simulink library "mympclib"  (R2020a)
settings: Solver=VariableStepAuto  StartTime=0.0  StopTime=10.0  RelTol=1e-3
values from neighbouring files (symbols this model uses):
  Ts = 0.01    [calcCTSyetem.m]
undefined symbols (not defined in the file or in its folder): params, sysm
settings Model: Creator=kohei  LastModifiedBy=kohei

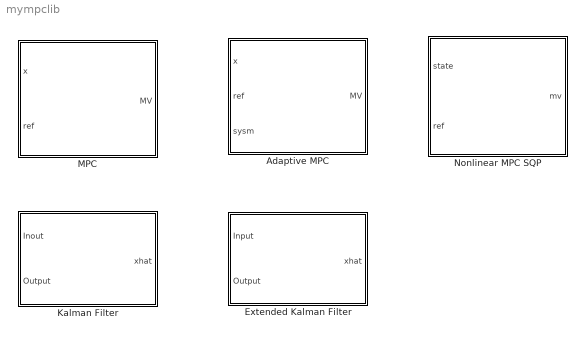
== system mympclib ==
  Adaptive MPC : Subsystem  TreatAsAtomicUnit=on  mask(Adaptive Model Predictive Control){params=params, numState=1, numRef=1, numMV=1, Ts=Ts, enableDist=off, numDist=1, enableSlack=off, enableStatus=off, enableMVseq=off}
      mask prompts: params "MPC Parameters"; numState "Dimension of State"; numRef "Dimension of Reference"; numMV "Dimension of Input"; Ts "Sampling time"; enableDist "Enable Disturbance Input"; numDist "Dimension of Disturbance"; enableSlack "Enable Slack Output"; enableStatus "Enable Status Output"; enableMVseq "Enable MVseq Output"
      mask help:
      | This is the Adaptive MPC (AMPC) Controller.
      | AMPC calculates the QP problem based on the linear plant model.
      | If you want to see the description, please push the help button.
      mask init:
      | numDist = initMaskPortMPC(numDist,enableDist,enableSlack,enableStatus,enableMVseq,'Adaptive MPC');
      | [params,~] = initMaskMPC(params,[],numState,numRef,numMV,numDist,'Adaptive MPC');
      | index = numState*params.PredictiveHorizon;
      | index2 = numMV*params.ControlHorizon;
      | index3 = numRef*params.PredictiveHorizon;
      | index4 = numMV*params.ControlHorizon+1;
      | index5 = 4*(numMV*params.ControlHorizon)+2*(numRef*params.PredictiveHorizon)+1;
      mask Help:
      | This block is the Adaptive MPC Controller.
      | AMPC calculates the QP problem based on the linear plant model.
      | 
      | >>Optimization formulation
      | -------------------------------------------------------------------------------------------------------------------------------------------------------------------
      | This MPC is formulated based on the next QP optimization.
      | 
      | J = 0.5 * ( (y - yref)'*Q*(y - yref) + du'*R*du + rho*slack^2 )
      | 
      | Subject to :
      | umin <= u <= umax
      | dumin <= du <= dumax
      | ymin - slack*vmin <= y <= ymax + slack*vmax
      | skack >= 0
      | 
      | One slack varable is introduced for relaxing the output constraint.
      | The vmin and vmax are the tunable parameter for relaxation which is able to specified by MPC parameter structure as "params.softConstRelaxation".
      | Please read the " Details of the parameter sturucture "params" and "sysm" ".
      | -------------------------------------------------------------------------------------------------------------------------------------------------------------------
      | 
      | >> Model Structure
      | -------------------------------------------------------------------------------------------------------------------------------------------------------------------
      | This block supports the discrete plant system as shown bellow:
      | Uppercase is indicated the Nominal value, Lowercase with 'd' suffix is indicated the perturbation.
      | 
      | State : x = X + dx
      | MV : u = U + du
      | Measurement Disturbance(MD) : md = MD + dmd
      | Output Value : y = Y +dy (dy = C*dx)
      | 
      | Model formulation :
      | dx(k+1) = A*dx(k)+ B*du(k) + Bd*dmd(k) + f0
      | y(K) = C*dx(K) + Y
      | 
      | Note : The direct feedthrough term "D" is not considered in this system.
      |           "f0" is the nominal value of the system at the operation point.
      | 
      | The plant model is streamed from the Input port "sysm" which is the Bus signal.
      | You need to define the Bus object named "sysBus" which includes A, B, Bd, C, f0 vector/matrix and the operation point of state, input, disturbance and output.
      | -------------------------------------------------------------------------------------------------------------------------------------------------------------------
      | 
      | >>Parameter
      | -------------------------------------------------------------------------------------------------------------------------------------------------------------------
      | The MPC parameter must be defined as structure variable.
      | And you must need to clarify the each dimension of "state", "ref", and "Input" and the Sampling time through mask dialog.
      | 
      | This block has four input ports "state", "ref", "md" and "sysm".
      | Where "n" is the order of state, "l" is the order of output value (OV), "m" is the order of manipulated variable (MV) and "nd" is the order of measurement disturbance (MD).
      | "state" : State variable of plant model (n×1)
      | "ref" : Reference for OV  (l×1)
      | "md" : Measurement Disturbance (nd×1)
      | "sysm" : Bus signal which includes the predictive model. The structuer of the Bus object is shown bellow :
      | 
      | sysm.A : A matrix
      | sysm.B : B matrix for MV
      | sysm.Bd : B matrix for MD
      | sysm.C : C matrix
      | sysm.U : Operation point of MV, Defalt : zeros(m,1)
      | sysm.MD : Operation point of MD, Default : zeros(nd,1)
      | sysm.Y : Operation point of OV, Default : zeros(l,1)
      | sysm.X : Operation point of state, Default : zeros(n,1)
      | sysm.f0: Operation point of system, Default : zeros(n,1)
      | 
      | You can create a Bus object automatically by uisng the API "createSysBusObject".
      | The API has four arguments 'n, m, nd, l'.
      | Example :
      | >sysBus = createSysBusObject(n,m,nd,l)
      | 
      | The output is four "mv" , "slack", "status" and "mvseq".
      | "mv" : Manipulated Variable which is optimized by MPC. (m×1)
      | "slack" : Slack variable for softening OV constrain. This value must be grater than 0 (>= 0).
      |              If the value is grater than 0, the OV constraint is softed to avoid infeasibe.
      | "status" : Status is for seeing whether or not feasible . If the value is "1", it means feasible, on the other hand the value is 0, it means infeasible.
      |                When the status is "0", the MPC applies a last MV for current step.
      | "mvseq": Sequence value of MV for futuer
      | -------------------------------------------------------------------------------------------------------------------------------------------------------------------
      | 
      | >>Solver
      | -------------------------------------------------------------------------------------------------------------------------------------------------------------------
      | You can choose two types solver for solving the QP.
      | First is the "Active set".
      | Second is the "Interior Point Method".
      | 
      | The Active set is appropriate to optimization class for small or middle size.
      | The Interior Point Method is appropriate to optimization class for large size.
      | 
      | Both default max iteration number is 50.
      | -------------------------------------------------------------------------------------------------------------------------------------------------------------------
      | 
      | >>Details of the parameter sturucture "params" and "sysm"
      | -------------------------------------------------------------------------------------------------------------------------------------------------------------------
      | The MPC parameter sturucture "params" must be configured as shown bellow :
      | Where "n" is the order of state, "l" is the order of OV, "m" is the order of MV and the "nd" is the order of MD.
      | 
      | params.Q : Weight of OV (l×l) , Default : Unit matrix
      | params.R : Weight of MV (m×m), Default : Unit matrix
      | params.PredictiveHorizon : Predictive horizon (Scalar), Default : 10
      | params.Controlhorizon : Control Horizon (Scalar), Default : 5
      | params.MV_max : MV max (m×1), Default : 999
      | params.MV_min : MV min (m×1), Default :  -999
      | params.dMV_max : Rate of MV max (m×1), Default : 999
      | params.dMV_min : Rate of MV min(m×1), Default : -999
      | params.OV_max : Rate of OV max (l×1), Default : 999
      | params.OV_min : Rate of OV min (l×1), Default : -999
      | params.rho : Weight of slack variable (Scalar), Default : 10^4
      | params.softConstRelaxation : Constant for OV relaxation by slack variable (l×1), Default : ones(l,1)
      | params.MV_scalefactor : Scale gain for MV (m×1), Default : ones(m,1)
      | params.OV_scalefactor : Scale gain for OV (l×1), Default : ones(m,1)
      | params.MD_scalefactor : Scale gain for MD (nd×1), Default : ones(m,1)
      | params.initialconditionMV : Initial value for MV (m×1), Default : ones(m,1)
      | params.SolverType :Scalar 1:= Active Set, 2:= Interior Point Method, Default : 1 (Active set)
      | params.IterationMax : Max iteration number of the QP solver, Default : 50
      | -------------------------------------------------------------------------------------------------------------------------------------------------------------------
      | 
      | >>Code generation
      | -------------------------------------------------------------------------------------------------------------------------------------------------------------------
      | Yes, support. If you have Simulink Coder and Embedded Coder, the implementation code can be generated from this block.
      | -------------------------------------------------------------------------------------------------------------------------------------------------------------------
      mask Callback enableDist:
      | enab = get_param(gcb,'enableDist');
      | 
      | % Set the 'MaskVisibilities' property for each parameters
      | if strcmp(enab,'on')
      |     set_param(gcb,'MaskVisibilities',{'on','on','on','on','on','on','on','on','on','on'});
      | else
      |     set_param(gcb,'MaskVisibilities',{'on','on','on','on','on','on','off','on','on','on'});
      | end
      mask Display:
      | fprintf('Adaptive MPC')
      | port_label('Output', 1, 'mv')
      | port_label('Input', 1, 'state')
      | port_label('Input', 2, 'ref')
      | port_label('Input', 3, 'sysm')
  Extended Kalman Filter : Subsystem  TreatAsAtomicUnit=on  mask(Extended Kalman filter){stateFunction=0, jacobianStateFunction=0, measurementFunction=0, jacobianMeasurmentFunction=0, Bv=0, Q=0, R=0, xhat0=0, P0=0, Ts=0, numState=0, numOutput=0, enableP=off, enableG=off}
      mask prompts: stateFunction "State Function"; jacobianStateFunction "Jacobian for the State Function"; measurementFunction "Measurment Function"; jacobianMeasurmentFunction "Jacobian for the Measurement Function"; Bv "Matrix for System noise v"; Q "Covariance matrix Q for system noise v"; R "Covariance matrix R for measurement noise w"; xhat0 "Initial value for xhat which is column vector"; P0 "Initial value for covariance matrix P"; Ts "Sampling time Ts"; numState "Order of state"; numOutput "Order of output"; enableP "Enable Covariance Marix output"; enableG "Enable Kalman Gain Matrix"
      mask help: This is the Extended Kalman filter(EKF) block.
      mask init:
      | p = initMaskEKF(stateFunction,measurementFunction,jacobianStateFunction,jacobianMeasurmentFunction);
      | initMaskPortKF(enableP,enableG,'EKF')
      mask Help:
      | This is the Extended Kalman filter(EKF) block.
      | Some parametrs are set through the mask diagram.
      | This block has two inputs named "Input" and "Output".
      | And it has three outputs named "xhat (Estimated state)", "P (Covariance matrix )" and "G (Kalman gain matrix )".
      | 
      | Support Formulation of EKF :
      | x(k+1) = f(x(k),u(k)) + Bv*v(k)
      | y(k) = h(x(k),u(k)) + w(k)
      | 
      | n : Order of state
      | m : Order of input
      | l : Order of output
      | 
      | f : Nonlinear dynamics function (n,1)
      | h : Nonlinear measurement function (l,1)
      | Bv : Gain matrix Bv for system noise v (n,n)
      | x : State (n,1)
      | u : Input (m,1)
      | v: System noise (n,1)
      | y : Output (l,1)
      | w : Measurement noise (l,1)
      | 
      | You need to prepare four MATLAB function and put them on the current folder or the MATLAB path.
      | Kind of the MATLAB function :
      | 
      | >Nonlinear discrete state function
      | 
      | >Jacobian of the Nonlinear state function about the state x with operate conditions x0 and u0.
      | 
      | >Nonlinear measurement function
      | 
      | >Jacobian of the Nonlinear measurement function about the state x with operate conditions x0 and u0.
      | 
      | Where, the above functions must be accepted three arguments x(state), u(input) and Ts(sampling time), and one output.
      | The order of three arguments has to be put as state, input and sampling time such like a below:
      | 
      | function out = fcn(x, u, Ts)
      | 
      | You have to set these function names through this mask dialog as the character array  by using sigle quotation.
      mask Display:
      | fprintf('Extended\n Kalman Filter')
      | port_label('Output', 1, 'xhat')
      | port_label('Input', 1, 'Input')
      | port_label('Input', 2, 'Output')
  Kalman Filter : Subsystem  TreatAsAtomicUnit=on  mask(Kalman filter){A=0, Bu=0, Bv=0, C=0, Q=0, R=0, xhat0=0, P0=0, Ts=0, enableP=off, enableG=off}
      mask prompts: A "System matrix A"; Bu "Input matrix Bu"; Bv "System noise matrix Bv"; C "Measurement matrix C"; Q "Covariance matrix for System noise v"; R "Covariance matrix for Measurement noise w"; xhat0 "Initial value for xhat which is column vector"; P0 "Initial value for covariance matrix P"; Ts "Sampling time Ts"; enableP "Enable Covariance Marix output"; enableG "Enable Kalman Gain Matrix"
      mask help: This is the LTI Kalman filter block.
      mask init:
      | initMaskPortKF(enableP,enableG,'KF')
      mask Help:
      | This is the LTI Kalman filter block.
      | All parametrs are set through the mask diagram.
      | This block has two inputs named "Input" and "Output".
      | And it has three outputs named "xhat (Estimated state)", "P (Covariance matrix )" and "G (Kalman gain matrix )".
      | 
      | Support Formulation of Kalman filter :
      | x(k+1) = A*x(k) + Bu*u(k) + Bv*v(k)
      | y(k) = C*x(k) + w(k)
      | 
      | A : System matrix A for state
      | Bu : System matrix Bu for input u
      | Bv : Gain matrix Bv for system noise v
      | C : System matrix C for output
      | x : State
      | u : Input
      | v : System noise
      | y : Output
      | w : Measurement noise
      mask Display:
      | fprintf('Kamlman Filter')
      | port_label('Output', 1, 'xhat')
      | port_label('Input', 1, 'Input')
      | port_label('Input', 2, 'Output')
  MPC : Subsystem  TreatAsAtomicUnit=on  mask(Model Predictive control){params=params, sysm=sysm, numState=1, numRef=1, numMV=1, Ts=Ts, enableDist=off, numDist=1, enableSlack=off, enableStatus=off, enableMVseq=off}
      mask prompts: params "MPC Parameters"; sysm "Control system"; numState "Dimension of State"; numRef "Dimension of Reference"; numMV "Dimension of MV"; Ts "Sampling time"; enableDist "Enable Disturbance Input"; numDist "Dimension of Disturbance"; enableSlack "Enable Slack Output"; enableStatus "Enable Status Output"; enableMVseq "Enable MVseq Output"
      mask help:
      | This is the MPC Controller.
      | MPC calculates the QP problem based on the linear plant model.
      | If you want to see the description, please push the help button.
      mask init:
      | numDist = initMaskPortMPC(numDist,enableDist,enableSlack,enableStatus,enableMVseq,'MPC');
      | [params,sysm] = initMaskMPC(params,sysm,numState,numRef,numMV,numDist,'MPC');
      | index = numState*params.PredictiveHorizon;
      | index2 = numMV*params.ControlHorizon;
      | index3 = numRef*params.PredictiveHorizon;
      | index4 = numMV*params.ControlHorizon+1;
      | index5 = 4*(numMV*params.ControlHorizon)+2*(numRef*params.PredictiveHorizon)+1;
      mask Help:
      | This block is the MPC Controller.
      | MPC calculates the QP problem based on the linear plant model.
      | 
      | >>Optimization formulation
      | -------------------------------------------------------------------------------------------------------------------------------------------------------------------
      | This MPC is formulated based on the next QP optimization.
      | 
      | J = 0.5 * ( (y - yref)'*Q*(y - yref) + du'*R*du + rho*slack^2 )
      | 
      | Subject to :
      | umin <= u <= umax
      | dumin <= du <= dumax
      | ymin - slack*vmin <= y <= ymax + slack*vmax
      | skack >= 0
      | 
      | One slack varable is introduced for releaxing the output constraint.
      | The vmin and vmax are tunable parameters for relaxation which are specified by the MPC parameter structure as "params.softConstRelaxation".
      | Please read the " Details of the parameter sturucture "params" and "sysm" ".
      | -------------------------------------------------------------------------------------------------------------------------------------------------------------------
      | 
      | 
      | >> Model Structure
      | -------------------------------------------------------------------------------------------------------------------------------------------------------------------
      | This block supports the discrete plant system as shown bellow:
      | Uppercase is indicated the Nominal value, Lowercase with 'd' suffix is indicated the perturbation.
      | 
      | State : x = X + dx
      | MV : u = U + du
      | Measurement Disturbance(MD) : md = MD + dmd
      | Output Value : y = Y +dy (dy = C*dx)
      | 
      | Model formulation :
      | dx(k+1) = A*dx(k)+ B*du(k) + Bd*dmd(k) + f0
      | y(K) = C*dx(K) + Y
      | 
      | Note : The direct feedthrough term "D" is not considered in this system.
      |           "f0" is the nominal value of the system at the operation point.
      | -------------------------------------------------------------------------------------------------------------------------------------------------------------------
      | 
      | 
      | >>Parameter
      | -------------------------------------------------------------------------------------------------------------------------------------------------------------------
      | The MPC parameter and the Control system must be defined as a structure variable.
      | The Sampling time must be set through mask dialog.
      | 
      | This block has three input ports "state", "ref" and "md".
      | Where, "n" is the order of state, "l" is the order of Output value (OV),  "m" is the order of Manipulated variable (MV) and "nd" is the order of measurment disturbance (MD).
      | "state" : State variable of plant model (n×1)
      | "ref" : Reference for OV  (l×1)
      | "md" : Measurement Disturbance (nd×1)
      | 
      | The output is three "mv" , "slack" and "status".
      | "MV" : Manipulated Variable which is optimized by MPC. (m×1)
      | "slack" : Slack variable for softening OV constrain. This value must be grater than 0 (>= 0).
      |              If the value is grater than 0, the OV constraint is softed to avoid infeasibe.
      | "status" : Status is for seeing whether or not feasible. If the value is "1", it means feasible, on the other hand the value is "0", it means infeasible.
      |                When the status is "0", the MPC applies a last MV for current step.
      | "mvseq": Sequence value of MV for futuer
      | -------------------------------------------------------------------------------------------------------------------------------------------------------------------
      | 
      | >>Solver
      | -------------------------------------------------------------------------------------------------------------------------------------------------------------------
      | You can choose two types solver for solving the QP.
      | First is the "Active set".
      | Second is the "Interior Point Method".
      | 
      | The Active set is appropriate to optimization class for small or middle size.
      | The Interior Point Method is appropriate to optimization class for large size.
      | 
      | Both default max iteration number is 50.
      | -------------------------------------------------------------------------------------------------------------------------------------------------------------------
      | 
      | >>Details of the parameter sturucture "params" and "sysm"
      | -------------------------------------------------------------------------------------------------------------------------------------------------------------------
      | The MPC parameter sturucture "params" must be configured as shown bellow :
      | Where the "n" is the order of state, "l" is the order of OV, "m" is the order of MV and the "nd" is the order of MD.
      | 
      | params.Q : Weight of OV (l×l) , Default : Unit matrix
      | params.R : Weight of MV (m×m), Default : Unit matrix
      | params.PredictiveHorizon : Predictive horizon (Scalar), Default : 10
      | params.Controlhorizon : Control Horizon (Scalar), Default : 5
      | params.MV_max : MV max (m×1), Default : 999
      | params.MV_min : MV min (m×1), Default :  -999
      | params.dMV_max : Rate of MV max (m×1), Default : 999
      | params.dMV_min : Rate of MV min(m×1), Default : -999
      | params.OV_max : Rate of OV max (l×1), Default : 999
      | params.OV_min : Rate of OV min (l×1), Default : -999
      | params.rho : Weight of slack variable (Scalar), Default : 10^4
      | params.softConstRelaxation : Constant for OV relaxation by slack variable (l×1), Default : ones(l,1)
      | params.MV_scalefactor : Scale gain for MV (m×1), Default : ones(m,1)
      | params.OV_scalefactor : Scale gain for OV (l×1), Default : ones(m,1)
      | params.MD_scalefactor : Scale gain for MD (nd×1), Default : ones(m,1)
      | params.initialconditionMV : Initial value for MV (m×1), Default : ones(m,1)
      | params.SolverType :Scalar, 1:= Active Set, 2:= Interior Point Method, Default : 1 (Active set)
      | params.IterationMax : Max iteration number of the QP solver, Default : 50
      | 
      | The Control system sturucture "syms" must be includes bellow items :
      | sysm.A : A matrix
      | sysm.B : B matrix for MV
      | sysm.Bd : B matrix for MD
      | sysm.C : C matrix
      | sysm.U : Operation point of MV, Defalt : zeros(m,1)
      | sysm.MD : Operation point of MD, Default : zeros(nd,1)
      | sysm.Y : Operation point of OV, Default : zeros(l,1)
      | sysm.X : Operation point of state, Default : zeros(n,1)
      | sysm.f0: Operation point of system, Default : zeros(n,1)
      | -------------------------------------------------------------------------------------------------------------------------------------------------------------------
      | 
      | >>Code generation
      | -------------------------------------------------------------------------------------------------------------------------------------------------------------------
      | Yes, support. If you have Simulink Coder and Embedded Coder, the implementation code can be generated from this block.
      | -------------------------------------------------------------------------------------------------------------------------------------------------------------------
      mask Callback enableDist:
      | enab = get_param(gcb,'enableDist');
      | 
      | % Set the 'MaskVisibilities' property for each parameters
      | if strcmp(enab,'on')
      |     set_param(gcb,'MaskVisibilities',{'on','on','on','on','on','on','on','on','on','on','on'});
      | else
      |     set_param(gcb,'MaskVisibilities',{'on','on','on','on','on','on','on','off','on','on','on'});
      | end
      mask Display:
      | fprintf('MPC')
      | port_label('Output', 1, 'mv')
      | port_label('Input', 1, 'state')
      | port_label('Input', 2, 'ref')
  Nonlinear MPC SQP : Subsystem  TreatAsAtomicUnit=on  mask(Nonlinear Model Predictive Control){params=params, nx=0, ny=0, nu=0, Ts=0, enableDist=off, nd=0, enableSlack=off, enableStatus=off}
      mask prompts: params "MPC Parameters"; nx "Dimension of State"; ny "Dimension of Output"; nu "Dimension of Input"; Ts "Sampling time"; enableDist "Enable Disturbance Input"; nd "Dimension of Disturbance"; enableSlack "Enable Slack Output"; enableStatus "Enable Status Output"
      mask help:
      | This is the NMPC Controller.
      | Calculate the NP problem by using the fmincon solver with SQP.
      |
      | Note :
      | "fmincon" is a builtin command of the Optimization Toolbox.
      | You need to install this toolbox for run this block.
      |
      | If you want to see the description, please push the help button.
      mask init:
      | nd = initMaskPortNMPC(nd,enableDist,enableSlack,enableStatus,'SQP');
      | params = initMaskNMPC(params,nx,ny,nu,nd);
      | mv0 = params.initialconditionMV;
      | x0 = params.initialconditionState;
      | Hp = params.PredictiveHorizon;
      | Hc = params.ControlHorizon;
      | d0 = [kron(ones(Hc,1),mv0);0];
      mask Help:
      | This block is the Nonlinear MPC Controller.
      | Calculate the NP problem by using the fmincon solver with SQP.
      | Note : "fmincon" is a builtin command of the Optimization Toolbox. You need to install this toolbox for run this block.
      | 
      | >>Optimization formulation
      | -------------------------------------------------------------------------------------------------------------------------------------------------------------------
      | This MPC is formulated based on the next QP optimization.
      | 
      | J = 0.5 * ( (y - yref)'*Q*(y - yref) + u'*R*u + rho*slack^2 )
      | 
      | Subject to :
      | umin <= u <= umax
      | dumin <= du <= dumax
      | ymin - slack*vmin <= y <= ymax + slack*vmax
      | skack >= 0
      | 
      | One slack varable is introduced for relaxing the output constraint.
      | The vmin and vmax are the tunable parameter for relaxation which is able to specified by MPC parameter structure as "params.softConstRelaxation".
      | Please read the " Details of the parameter sturucture "params"' and "sysm" ".
      | -------------------------------------------------------------------------------------------------------------------------------------------------------------------
      | 
      | 
      | >> Model Structure
      | -------------------------------------------------------------------------------------------------------------------------------------------------------------------
      | This block supports the discrete nonlinear plant system as shown bellow:
      | 
      | Model formulation :
      | dx(k+1) = f( x(k), u(k) ,d(k) )
      | y(K) = h( x(k), u(k) )
      | 
      | The "f" is the state function and the "h" is the measurement function.
      | These are defined by MATLAB Function.
      | -------------------------------------------------------------------------------------------------------------------------------------------------------------------
      | 
      | >>Parameter
      | -------------------------------------------------------------------------------------------------------------------------------------------------------------------
      | The MPC parameter must be defined as structure variable.
      | And you must need to clarify the each dimension of "State", "Output", "Input" and Sampling time through mask dialog.
      | 
      | This block has three input ports "state", "ref", and "md".
      | Where "n" is the order of state, "l" is the order of output value (OV),  "m" is the order of manipulated variable (MV) and "nd" is the order of measurement disturbance (MD).
      | "state" : State variable of plant model (n×1)
      | "ref" : Reference for OV  (l×1)
      | "md" : Measurement Disturbance (nd×1)
      | 
      | The output is three "mv" , "slack", and "status".
      | "mv" : Manipulated Variable which is optimized by MPC. (m×1)
      | "slack" : Slack variable for softening OV constraint. This value must be grater than 0 (>= 0).
      |              If the value is grater than 0, the OV constraint is softed to avoid infeasibe solution.
      | "status" : Status is for seeing whether or not feasible. If the value is "1", it means feasible, on the other hand the value is 0, it means infeasible.
      |                When the value equals "0", the MPC applies a last MV for current step.
      | -------------------------------------------------------------------------------------------------------------------------------------------------------------------
      | 
      | >>Solver
      | -------------------------------------------------------------------------------------------------------------------------------------------------------------------
      | NMPC block is implemented by using the "fmincon".
      | And for solving NP problem, SQP algorithm is used.
      | The "fmincon" is builtin command of the Optimization Toolbox.
      | So, you need to install the toolbox in your machine.
      | Default max iteration number is 50 times.
      | -------------------------------------------------------------------------------------------------------------------------------------------------------------------
      | 
      | >>Details of the parameter sturucture "params".
      | -------------------------------------------------------------------------------------------------------------------------------------------------------------------
      | The MPC parameter sturucture "params" must be configured as shown bellow :
      | Where "n" is the order of state, "l" is the order of OV, "m" is the order of MV.
      | 
      | params.stateFunction : Function name for the state evolution
      | params.measurementFunction : Function name for the measurement
      | params.Q : Weight of OV (l×l) , Default : Unit matrix
      | params.R : Weight of MV (m×m), Default : Unit matrix
      | params.PredictiveHorizon : Predictive horizon (Scalar), Default : 10
      | params.Controlhorizon : Control Horizon (Scalar), Default : 5
      | params.MV_max : MV max (m×1), Default : 999
      | params.MV_min : MV min (m×1), Default :  -999
      | params.dMV_max : Rate of MV max (m×1), Default : 999
      | params.dMV_min : Rate of MV min(m×1), Default : -999
      | params.OV_max : Rate of OV max (l×1), Default : 999
      | params.OV_min : Rate of OV min (l×1), Default : -999
      | params.rho : Weight of slack variable (Scalar), Default : 10^4
      | params.softConstRelaxation : Constant for OV relaxation by slack variable (l×1), Default : ones(l,1)
      | params.MV_scalefactor : Scale gain for MV (m×1), Default : ones(m,1)
      | params.OV_scalefactor : Scale gain for OV (l×1), Default : ones(m,1)
      | params.initialconditionMV : Initial value for MV (m×1), Default : zeros(m,1)
      | params.initialconditionState : Initial value for State (n×1), Default : zeros(m,1)
      | params.IterationMax : Max iteration number of the solver, Default : 50
      | -------------------------------------------------------------------------------------------------------------------------------------------------------------------
      | 
      | >>Code generation
      | -------------------------------------------------------------------------------------------------------------------------------------------------------------------
      | Yes, support. If you have Simulink Coder and Embedded Coder, the implementation code can be generated from this block.
      | -------------------------------------------------------------------------------------------------------------------------------------------------------------------
      mask Callback enableStatus:
      | enab = get_param(gcb,'enableDist');
      | 
      | % Set the 'MaskVisibilities' property for each parameters
      | if strcmp(enab,'on')
      |     set_param(gcb,'MaskVisibilities',{'on','on','on','on','on','on','on','on','on'});
      | else
      |     set_param(gcb,'MaskVisibilities',{'on','on','on','on','on','on','off','on','on'});
      | end
      mask Display:
      | fprintf('Nonlinear MPC\nSQP')
      | port_label('Output', 1, 'mv')
      | port_label('Input', 1, 'state')
      | port_label('Input', 2, 'ref')

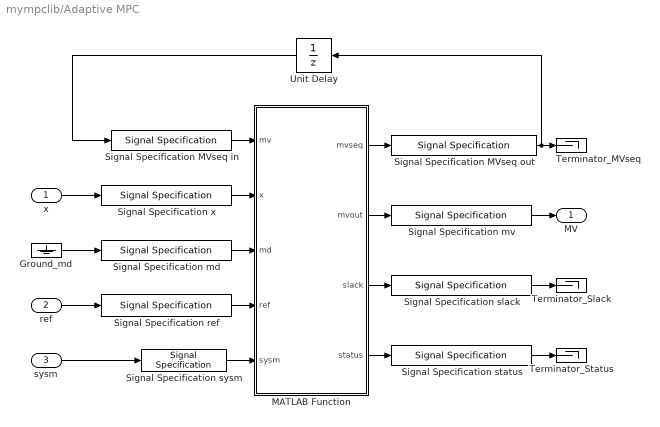
== system mympclib/Adaptive MPC ==
  x : Inport
  ref : Inport  Port=2
  sysm : Inport  Port=3
  Ground_md : Ground
  MATLAB Function : MATLAB Function  TreatAsAtomicUnit=on  SystemSampleTime=Ts
  Signal Specification MVseq in : SignalSpecification  OutDataTypeStr=double  Dimensions=index2  SampleTime=Ts
  Signal Specification MVseq out : SignalSpecification  OutDataTypeStr=double  Dimensions=index2  SampleTime=Ts
  Signal Specification md : SignalSpecification  OutDataTypeStr=double  Dimensions=numDist  SampleTime=Ts
  Signal Specification mv : SignalSpecification  OutDataTypeStr=double  Dimensions=numMV  SampleTime=Ts
  Signal Specification ref : SignalSpecification  OutDataTypeStr=double  Dimensions=numRef  SampleTime=Ts
  Signal Specification slack : SignalSpecification  OutDataTypeStr=double  Dimensions=1  SampleTime=Ts
  Signal Specification status : SignalSpecification  OutDataTypeStr=boolean  Dimensions=1  SampleTime=Ts
  Signal Specification sysm : SignalSpecification  SampleTime=Ts
  Signal Specification x : SignalSpecification  OutDataTypeStr=double  Dimensions=numState  SampleTime=Ts
  Terminator_MVseq : Terminator
  Terminator_Slack : Terminator
  Terminator_Status : Terminator
  Unit Delay : UnitDelay  InitialCondition=kron(ones(params.ControlHorizon,1) , params.initialconditionMV)  SampleTime=-1  HasFrameUpgradeWarning=on
  MV : Outport
  wires:
  MATLAB Function/3(slack) -> Signal Specification slack/1
  MATLAB Function/4(status) -> Signal Specification status/1
  x/1 -> Signal Specification x/1
  ref/1 -> Signal Specification ref/1
  Signal Specification x/1 -> MATLAB Function/2(x)
  Signal Specification md/1 -> MATLAB Function/3(md)
  Signal Specification ref/1 -> MATLAB Function/4(ref)
  sysm/1 -> Signal Specification sysm/1
  MATLAB Function/2(mvout) -> Signal Specification mv/1
  Signal Specification sysm/1 -> MATLAB Function/5(sysm)
  MATLAB Function/1(mvseq) -> Signal Specification MVseq out/1
  Unit Delay/1 -> Signal Specification MVseq in/1
  Signal Specification mv/1 -> MV/1
  Signal Specification MVseq in/1 -> MATLAB Function/1(mv)
  Signal Specification MVseq out/1 -> Unit Delay/1, Terminator_MVseq/1
  Signal Specification slack/1 -> Terminator_Slack/1
  Signal Specification status/1 -> Terminator_Status/1
  Ground_md/1 -> Signal Specification md/1

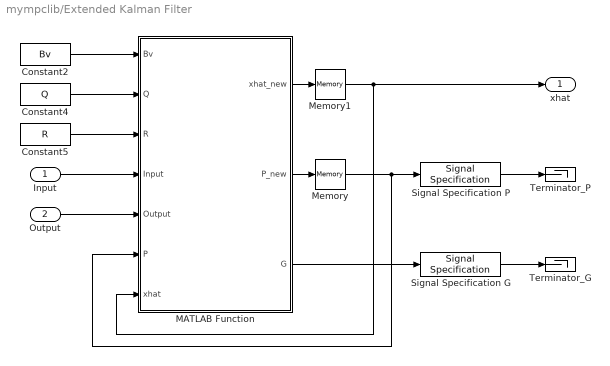
== system mympclib/Extended Kalman Filter ==
  Input : Inport
  Output : Inport  Port=2
  Constant2 : Constant  Value=Bv
  Constant4 : Constant  Value=Q
  Constant5 : Constant  Value=R
  MATLAB Function : MATLAB Function  TreatAsAtomicUnit=on  SystemSampleTime=Ts
  Memory : Memory  InitialCondition=P0  InheritSampleTime=on  LinearizeMemory=on  LinearizeAsDelay=on
  Memory1 : Memory  InitialCondition=xhat0  InheritSampleTime=on  LinearizeMemory=on  LinearizeAsDelay=on
  Signal Specification G : SignalSpecification  SampleTime=Ts
  Signal Specification P : SignalSpecification  SampleTime=Ts
  Terminator_G : Terminator
  Terminator_P : Terminator
  xhat : Outport
  wires:
  Constant2/1 -> MATLAB Function/1(Bv)
  MATLAB Function/3(G) -> Signal Specification G/1
  Constant5/1 -> MATLAB Function/3(R)
  Memory1/1 -> xhat/1, MATLAB Function/7(xhat)
  MATLAB Function/2(P_new) -> Memory/1
  MATLAB Function/1(xhat_new) -> Memory1/1
  Input/1 -> MATLAB Function/4(Input)
  Output/1 -> MATLAB Function/5(Output)
  Constant4/1 -> MATLAB Function/2(Q)
  Memory/1 -> Signal Specification P/1, MATLAB Function/6(P)
  Signal Specification P/1 -> Terminator_P/1
  Signal Specification G/1 -> Terminator_G/1

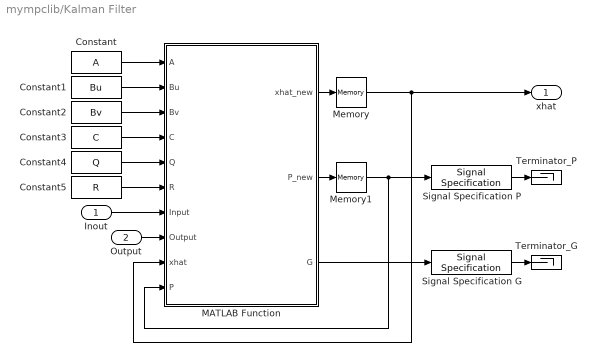
== system mympclib/Kalman Filter ==
  Inout : Inport
  Output : Inport  Port=2
  Constant : Constant  Value=A
  Constant1 : Constant  Value=Bu
  Constant2 : Constant  Value=Bv
  Constant3 : Constant  Value=C
  Constant4 : Constant  Value=Q
  Constant5 : Constant  Value=R
  MATLAB Function : MATLAB Function  TreatAsAtomicUnit=on  SystemSampleTime=Ts
  Memory : Memory  InitialCondition=xhat0  InheritSampleTime=on  LinearizeMemory=on  LinearizeAsDelay=on
  Memory1 : Memory  InitialCondition=P0  InheritSampleTime=on  LinearizeMemory=on  LinearizeAsDelay=on
  Signal Specification G : SignalSpecification  SampleTime=Ts
  Signal Specification P : SignalSpecification  SampleTime=Ts
  Terminator_G : Terminator
  Terminator_P : Terminator
  xhat : Outport
  wires:
  MATLAB Function/3(G) -> Signal Specification G/1
  Constant1/1 -> MATLAB Function/2(Bu)
  MATLAB Function/2(P_new) -> Memory1/1
  MATLAB Function/1(xhat_new) -> Memory/1
  Constant5/1 -> MATLAB Function/6(R)
  Inout/1 -> MATLAB Function/7(Input)
  Constant2/1 -> MATLAB Function/3(Bv)
  Constant3/1 -> MATLAB Function/4(C)
  Constant/1 -> MATLAB Function/1(A)
  Output/1 -> MATLAB Function/8(Output)
  Constant4/1 -> MATLAB Function/5(Q)
  Memory/1 -> MATLAB Function/9(xhat), xhat/1
  Memory1/1 -> MATLAB Function/10(P), Signal Specification P/1
  Signal Specification P/1 -> Terminator_P/1
  Signal Specification G/1 -> Terminator_G/1

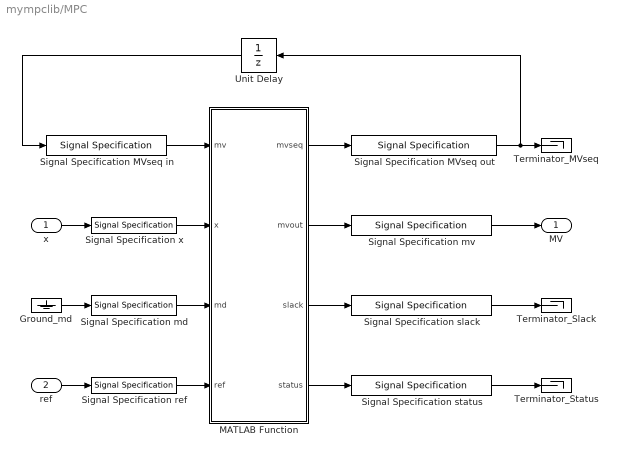
== system mympclib/MPC ==
  x : Inport
  ref : Inport  Port=2
  Ground_md : Ground
  MATLAB Function : MATLAB Function  TreatAsAtomicUnit=on  SystemSampleTime=Ts
  Signal Specification MVseq in : SignalSpecification  OutDataTypeStr=double  Dimensions=index2  SampleTime=Ts
  Signal Specification MVseq out : SignalSpecification  OutDataTypeStr=double  Dimensions=index2  SampleTime=Ts
  Signal Specification md : SignalSpecification  Dimensions=numDist  SampleTime=Ts
  Signal Specification mv : SignalSpecification  OutDataTypeStr=double  Dimensions=numMV  SampleTime=Ts
  Signal Specification ref : SignalSpecification  Dimensions=numRef  SampleTime=Ts
  Signal Specification slack : SignalSpecification  OutDataTypeStr=double  Dimensions=1  SampleTime=Ts
  Signal Specification status : SignalSpecification  OutDataTypeStr=boolean  Dimensions=1  SampleTime=Ts
  Signal Specification x : SignalSpecification  Dimensions=numState  SampleTime=Ts
  Terminator_MVseq : Terminator
  Terminator_Slack : Terminator
  Terminator_Status : Terminator
  Unit Delay : UnitDelay  InitialCondition=kron(ones(params.ControlHorizon,1) , params.initialconditionMV)  SampleTime=-1  HasFrameUpgradeWarning=on
  MV : Outport
  wires:
  Signal Specification ref/1 -> MATLAB Function/4(ref)
  Signal Specification md/1 -> MATLAB Function/3(md)
  Signal Specification x/1 -> MATLAB Function/2(x)
  ref/1 -> Signal Specification ref/1
  x/1 -> Signal Specification x/1
  MATLAB Function/4(status) -> Signal Specification status/1
  MATLAB Function/3(slack) -> Signal Specification slack/1
  MATLAB Function/2(mvout) -> Signal Specification mv/1
  Signal Specification MVseq in/1 -> MATLAB Function/1(mv)
  MATLAB Function/1(mvseq) -> Signal Specification MVseq out/1
  Signal Specification mv/1 -> MV/1
  Signal Specification MVseq out/1 -> Unit Delay/1, Terminator_MVseq/1
  Unit Delay/1 -> Signal Specification MVseq in/1
  Ground_md/1 -> Signal Specification md/1
  Signal Specification slack/1 -> Terminator_Slack/1
  Signal Specification status/1 -> Terminator_Status/1

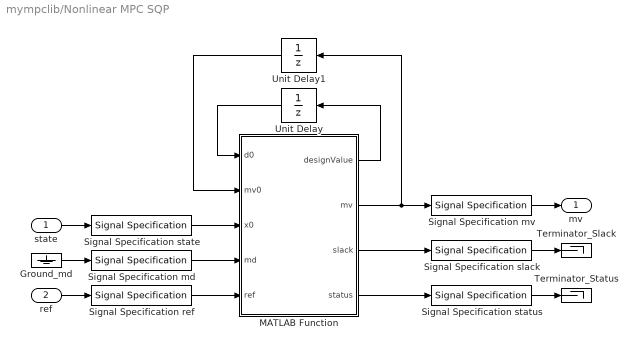
== system mympclib/Nonlinear MPC SQP ==
  state : Inport
  ref : Inport  Port=2
  Ground_md : Ground
  MATLAB Function : MATLAB Function  TreatAsAtomicUnit=on  SystemSampleTime=Ts
  Signal Specification md : SignalSpecification  OutDataTypeStr=double  Dimensions=nd  SampleTime=Ts
  Signal Specification mv : SignalSpecification  OutDataTypeStr=double  Dimensions=nu  SampleTime=Ts
  Signal Specification ref : SignalSpecification  OutDataTypeStr=double  Dimensions=ny  SampleTime=Ts
  Signal Specification slack : SignalSpecification  OutDataTypeStr=double  Dimensions=1  SampleTime=Ts
  Signal Specification state : SignalSpecification  OutDataTypeStr=double  Dimensions=nx  SampleTime=Ts
  Signal Specification status : SignalSpecification  OutDataTypeStr=boolean  Dimensions=1  SampleTime=Ts
  Terminator_Slack : Terminator
  Terminator_Status : Terminator
  Unit Delay : UnitDelay  InitialCondition=d0  SampleTime=Ts  HasFrameUpgradeWarning=on
  Unit Delay1 : UnitDelay  InitialCondition=mv0  SampleTime=Ts  HasFrameUpgradeWarning=on
  mv : Outport
  wires:
  state/1 -> Signal Specification state/1
  MATLAB Function/2(mv) -> Signal Specification mv/1, Unit Delay1/1
  MATLAB Function/1(designValue) -> Unit Delay/1
  Unit Delay/1 -> MATLAB Function/1(d0)
  ref/1 -> Signal Specification ref/1
  MATLAB Function/4(status) -> Signal Specification status/1
  MATLAB Function/3(slack) -> Signal Specification slack/1
  Unit Delay1/1 -> MATLAB Function/2(mv0)
  Signal Specification state/1 -> MATLAB Function/3(x0)
  Signal Specification md/1 -> MATLAB Function/4(md)
  Signal Specification ref/1 -> MATLAB Function/5(ref)
  Signal Specification mv/1 -> mv/1
  Ground_md/1 -> Signal Specification md/1
  Signal Specification slack/1 -> Terminator_Slack/1
  Signal Specification status/1 -> Terminator_Status/1

== matlab function mympclib/Nonlinear MPC SQP/MATLAB Function ==
  data: d0 input; mv0 input; designValue output; x0 input; md input; ref input; mv output; slack output; status output; params parameter; ny parameter; nu parameter; nx parameter
function [designValue,mv,slack,status] = fcn(d0,mv0,x0,md,ref,params,ny,nu,nx)
% Wraper for the nmpcfcn

% Initialization
designValue = zeros(length(d0),1,'like',d0);
mv = zeros(length(mv0),1,'like',mv0);
slack = zeros(1);
status = false;

[designValue,mv,slack,status] = nmpcfcn(d0,x0,mv0,md,ref,params,ny,nu,nx);
end
%EOF

== matlab function mympclib/Kalman Filter/MATLAB Function ==
  data: A input; xhat_new output; Bu input; Bv input; C input; Q input; R input; Input input; Output input; xhat input; P input; P_new output; G output
function [xhat_new,P_new,G] = fcn(A,Bu,Bv,C,Q,R,Input,Output,xhat,P)
%#codegen
% Wrapper function for Kalman filter function kf

% Initialization
n = size(A,1);
l = length(Output);
xhat_new = zeros(n,1);
P_new = zeros(n);
G = zeros(n,l);

% Call kf fucntion
[xhat_new,P_new,G] = kf(A,Bu,Bv,C,Q,R,Input,Output,xhat,P);
end
%EOF

== matlab function mympclib/MPC/MATLAB Function ==
  data: mvseq output; mv input; x input; mvout output; md input; ref input; slack output; status output boolean; params parameter; sysm parameter; index parameter size=1; index2 parameter size=1; index3 parameter size=1; index4 parameter size=1; index5 parameter size=1
function [mvseq,mvout,slack,status] = fcn(mv,x,md,ref,params,sysm,index,index2,index3,index4,index5)
% Wrapper of "mpcfcn"
% x:Output value(OV)
% d:Disturbance
% ref:Reference for OV
% sysm:Construnstion of system(A,B,C,D)
% params:MPC parameter constructs
% Dimenstions of each matrix:
% index = n*Hp
% index2 = m*Hc
% index3 = l*Hp
% index4 = (m*Hc)+1
% index5 = (4*index2)+(2*index3)+1
% Initlialization of outputs

% coder.extrinsic('mpcfcn');

% Initlialization of outputs
m = size(sysm.B,2);
slack = zeros(1);
status = false;
mvseq = zeros(index2,1);
mvout = zeros(m,1);

% Call mpcfcn
[mvopt,slack,status] = mpcfcn(x,mv,md,ref,sysm,params,index,index2,index3,index4,index5);
mvout = mvopt(1:m,1);
mvseq = mvopt;
%EOF

== matlab function mympclib/Adaptive MPC/MATLAB Function ==
  data: mvseq output; mv input; x input; mvout output; md input; ref input; slack output; status output boolean; params parameter; sysm input; index parameter size=1; index2 parameter size=1; index3 parameter size=1; index4 parameter size=1; index5 parameter size=1
function [mvseq,mvout,slack,status] = fcn(mv,x,md,ref,params,sysm,index,index2,index3,index4,index5)
% Wrapper of "mpcfcn"
% x:Output value(OV)
% d:Disturbance
% ref:Reference for OV
% sysm:Construnstion of system(A,B,C,D)
% params:MPC parameter constructs
% Dimenstions of each matrix:
% index = n*Hp
% index2 = m*Hc
% index3 = l*Hp
% index4 = (m*Hc)+1
% index5 = (4*index2)+(2*index3)+1

% Initlialization of outputs
m = size(sysm.B,2);
slack = zeros(1);
status = false;
mvseq = zeros(index2,1);
mvout = zeros(m,1);

% Call mpcfcn
[mvopt,slack,status] = mpcfcn(x,mv,md,ref,sysm,params,index,index2,index3,index4,index5);
mvout = mvopt(1:m,1);
mvseq = mvopt;
%EOF

== matlab function mympclib/Extended Kalman Filter/MATLAB Function ==
  data: xhat_new output; Bv input; Q input; R input; Input input; Output input; P input; xhat input; P_new output; G output; numState parameter; numOutput parameter; Ts parameter; p parameter
function [xhat_new,P_new,G] = fcn(Bv,Q,R,Input,Output,P,xhat,numState,numOutput,Ts,p)
%#codegen
% Wrapper function for Extended Kalman filter function ekf

% Initialization
n = numState;
l = numOutput;
xhat_new = zeros(n,1);
P_new = zeros(n);
G = zeros(n,l);

% Function handle
f = str2func(p.stateFunction);
h = str2func(p.measurementFunction);
A = str2func(p.jacobianStateFunction);
C = str2func(p.jacobianOfMeasurementFunction);

% Call kf fucntion
[xhat_new,P_new,G] = ekf(f,h,A,C,Bv,Q,R,Input,Output,xhat,P,Ts);
end
%EOF
